simulink model "LoFT_Example3"  (R2024b)
settings: Solver=ode4  StartTime=0.0  StopTime=300  FixedStep=simu.dt  RelTol=1e-3
undefined symbols (not defined in the file): body, circtime, Communication, D1, Delta, irkb, line, LoFT, p0, Pn, s, simu, trip_time, Turbwind, waves, wind
libraries: simulink x350, spsThreePhaseVIMeasurementLib x41, spsThreePhasePISectionLineLib x34, spsThreePhaseParallelRLCLoadLib x21, spsThreePhaseTransformerTwoWindingsLib x14, spsLoadFlowBusLib x10, spsThreePhaseDynamicLoadLib x9, spsSynchronousMachinepuStandardLib x7, spsExcitationSystemLib x7, spsSteamTurbineandGovernorLib x7, spsGenericPowerSystemStabilizerLib x7, spsMultiBandPowerSystemStabilizerLib x7
(part 45 of 49)

== system LoFT_Example3/FOWT System/Subsystem7/FOWT9/Aerodynamics and Local Control Systems/Local Control Systems/Subsystem2 ==
  GenTorq : Inport
  BldPitch : Inport  Port=2
  Constant3 : Constant  Value=-Controller.torqueMax
  Gain 1 : Gain  Gain=Controller.SPS_kb/deg2rad(30)
  Gain 2 : Gain  Gain=Controller.omegaMax
  Gain 3 : Gain  Gain=-Controller.SPS_kt/Controller.torqueMax
  Sum5 : Sum  Inputs=|+-
  Sum6 : Sum  Inputs=|+-
  Delta_omega_g : Outport
  wires:
  Sum6/1 -> Gain 2/1
  Gain 1/1 -> Sum6/1
  Constant3/1 -> Sum5/2
  Gain 3/1 -> Sum6/2
  Sum5/1 -> Gain 3/1
  Gain 2/1 -> Delta_omega_g/1
  BldPitch/1 -> Gain 1/1
  GenTorq/1 -> Sum5/1

== system LoFT_Example3/FOWT System/Subsystem7/FOWT9/Aerodynamics and Local Control Systems/Local Control Systems/wind speed estimator ==
  In1 : Inport
  Discrete Filter : DiscreteFilter  Numerator=Controller.F.Wind.b  Denominator=Controller.F.Wind.a  InitialStates=2000
  Out1 : Outport
  wires:
  Discrete Filter/1 -> Out1/1
  In1/1 -> Discrete Filter/1

== system LoFT_Example3/Onshore grid/Onshore Grid/Subsystem/SG1/Regulators1/Turbine  & Excitation Regulators Mac2 ==
  Pref : Inport
  Vref : Inport  Port=2
  Vd : Inport  Port=3
  Vq : Inport  Port=4
  w : Inport  Port=5
  Pe : Inport  Port=6
  Add : Sum  Inputs=+-
  Excitation System : spsExcitationSystemLib/Excitation System  tr=20e-3  reg=[ 300, 0.001 ]  exc=[ 1, 0 ]  tgr=[ 0, 0 ]  damp=[ 0.001, 0.1 ]  sat=[ 0, 0 ]  lim=[ -11.5, 11.5, 0 ]  v0=[1 1.43]
  STG : spsSteamTurbineandGovernorLib/Steam Turbine and Governor  gentype=Tandem-compound (single mass)  reg1="[ 20  0.05    0 ]"  reg2="[ 0.001  0.15 ]"  reg3="[ -0.1  0.1  0  4.496 ]"  N=60*50  turb1="[ 0  10   3.3   0.5   ]"  turb2="[   0   0.36    0.36   0.28   ]"  HA="[ 0.046  1.430  1.465   0.192 ]"  KA="[ 90.44  53.88  64.59   62.94  ]"  DA="[ 0.0115  0.3575  0.3663   0.0137  ]"  ini1=1  ini2=[0.779316,-31.4247]
  Stabilisateur : Subsystem
  Terminator : Terminator
  Terminator1 : Terminator
  Terminator2 : Terminator
  wref : Constant
  wref1 : Constant
  Pm : Outport  VectorParamsAs1DForOutWhenUnconnected=off
  Vf : Outport  Port=2  VectorParamsAs1DForOutWhenUnconnected=off
  wires:
  Stabilisateur/1(Stab) -> Excitation System/4
  Add/1 -> STG/4, Stabilisateur/3(dw)
  wref1/1 -> Add/2
  Vd/1 -> Excitation System/2
  Vq/1 -> Excitation System/3
  w/1 -> STG/3, Add/1
  wref/1 -> STG/1
  Vref/1 -> Excitation System/1
  Pref/1 -> STG/2
  Pe/1 -> Stabilisateur/2(Pe)
  Excitation System/1 -> Vf/1
  STG/4 -> Stabilisateur/1(Pm), Pm/1
  STG/3 -> Terminator/1
  STG/2 -> Terminator1/1
  STG/1 -> Terminator2/1

== system LoFT_Example3/Onshore grid/Onshore Grid/Subsystem/SG2/Regulators2/Turbine  & Excitation Regulators Mac2 ==
  Pref : Inport
  Vref : Inport  Port=2
  Vd : Inport  Port=3
  Vq : Inport  Port=4
  w : Inport  Port=5
  Pe : Inport  Port=6
  Add : Sum  Inputs=+-
  Add1 : Sum
  Excitation System : spsExcitationSystemLib/Excitation System  tr=20e-3  reg=[ 300, 0.001 ]  exc=[ 1, 0 ]  tgr=[ 0, 0 ]  damp=[ 0.001, 0.1 ]  sat=[ 0, 0 ]  lim=[ -11.5, 11.5, 0 ]  v0=[1 1.43]
  STG : spsSteamTurbineandGovernorLib/Steam Turbine and Governor  gentype=Tandem-compound (single mass)  reg1="[ 20  0.05    0 ]"  reg2="[ 0.001  0.15 ]"  reg3="[ -0.1  0.1  0  4.496 ]"  N=60*50  turb1="[ 0  10   3.3   0.5   ]"  turb2="[   0   0.36    0.36   0.28   ]"  HA="[ 0.046  1.430  1.465   0.192 ]"  KA="[ 90.44  53.88  64.59   62.94  ]"  DA="[ 0.0115  0.3575  0.3663   0.0137  ]"  ini1=0.54  ini2=[0.779316,-31.4247]
  Stabilisateur : Subsystem
  Terminator : Terminator
  Terminator1 : Terminator
  Terminator2 : Terminator
  wref : Constant
  wref1 : Constant
  Pm : Outport  VectorParamsAs1DForOutWhenUnconnected=off
  Vf : Outport  Port=2  VectorParamsAs1DForOutWhenUnconnected=off
  wires:
  Stabilisateur/1(Stab) -> Excitation System/4
  Add/1 -> STG/4, Stabilisateur/3(dw)
  wref1/1 -> Add/2
  Vd/1 -> Excitation System/2
  Vq/1 -> Excitation System/3
  w/1 -> STG/3, Add/1
  wref/1 -> STG/1
  Vref/1 -> Excitation System/1
  Pref/1 -> STG/2
  Pe/1 -> Stabilisateur/2(Pe)
  Excitation System/1 -> Vf/1
  STG/4 -> Stabilisateur/1(Pm), Add1/2
  STG/3 -> Terminator/1
  STG/2 -> Terminator1/1
  STG/1 -> Terminator2/1
  Add1/1 -> Pm/1

== system LoFT_Example3/Onshore grid/Onshore Grid/Subsystem/SG4/Regulators4/Turbine  & Excitation Regulators Mac2 ==
  Pref : Inport
  Vref : Inport  Port=2
  Vd : Inport  Port=3
  Vq : Inport  Port=4
  w : Inport  Port=5
  Pe : Inport  Port=6
  Add : Sum  Inputs=+-
  Add1 : Sum
  Excitation System : spsExcitationSystemLib/Excitation System  tr=20e-3  reg=[ 300, 0.001 ]  exc=[ 1, 0 ]  tgr=[ 0, 0 ]  damp=[ 0.001, 0.1 ]  sat=[ 0, 0 ]  lim=[ -11.5, 11.5, 0 ]  v0=[1 1.43]
  STG : spsSteamTurbineandGovernorLib/Steam Turbine and Governor  gentype=Tandem-compound (single mass)  reg1="[ 20  0.05    0 ]"  reg2="[ 0.001  0.15 ]"  reg3="[ -0.1  0.1  0  4.496 ]"  N=60*50  turb1="[ 0  10   3.3   0.5   ]"  turb2="[   0   0.36    0.36   0.28   ]"  HA="[ 0.046  1.430  1.465   0.192 ]"  KA="[ 90.44  53.88  64.59   62.94  ]"  DA="[ 0.0115  0.3575  0.3663   0.0137  ]"  ini1=0.54  ini2=[0.779316,-31.4247]
  Stabilisateur : Subsystem
  Terminator : Terminator
  Terminator1 : Terminator
  Terminator2 : Terminator
  wref : Constant
  wref1 : Constant
  Pm : Outport  VectorParamsAs1DForOutWhenUnconnected=off
  Vf : Outport  Port=2  VectorParamsAs1DForOutWhenUnconnected=off
  wires:
  Stabilisateur/1(Stab) -> Excitation System/4
  Add/1 -> STG/4, Stabilisateur/3(dw)
  wref1/1 -> Add/2
  Vd/1 -> Excitation System/2
  Vq/1 -> Excitation System/3
  w/1 -> STG/3, Add/1
  wref/1 -> STG/1
  Vref/1 -> Excitation System/1
  Pref/1 -> STG/2
  Pe/1 -> Stabilisateur/2(Pe)
  Excitation System/1 -> Vf/1
  STG/4 -> Stabilisateur/1(Pm), Add1/2
  STG/3 -> Terminator/1
  STG/2 -> Terminator1/1
  STG/1 -> Terminator2/1
  Add1/1 -> Pm/1

== system LoFT_Example3/Onshore grid/Onshore Grid/Subsystem/SG5/Regulators5/Turbine  & Excitation Regulators Mac2 ==
  Pref : Inport
  Vref : Inport  Port=2
  Vd : Inport  Port=3
  Vq : Inport  Port=4
  w : Inport  Port=5
  Pe : Inport  Port=6
  Add : Sum  Inputs=+-
  Excitation System : spsExcitationSystemLib/Excitation System  tr=20e-3  reg=[ 300, 0.001 ]  exc=[ 1, 0 ]  tgr=[ 0, 0 ]  damp=[ 0.001, 0.1 ]  sat=[ 0, 0 ]  lim=[ -11.5, 11.5, 0 ]  v0=[1 1.43]
  STG : spsSteamTurbineandGovernorLib/Steam Turbine and Governor  gentype=Tandem-compound (single mass)  reg1="[ 20  0.05    0 ]"  reg2="[ 0.001  0.15 ]"  reg3="[ -0.1  0.1  0  4.496 ]"  N=60*50  turb1="[ 0  10   3.3   0.5   ]"  turb2="[   0   0.36    0.36   0.28   ]"  HA="[ 0.046  1.430  1.465   0.192 ]"  KA="[ 90.44  53.88  64.59   62.94  ]"  DA="[ 0.0115  0.3575  0.3663   0.0137  ]"  ini1=0.508  ini2=[0.779316,-31.4247]
  Stabilisateur : Subsystem
  Terminator : Terminator
  Terminator1 : Terminator
  Terminator2 : Terminator
  wref : Constant
  wref1 : Constant
  Pm : Outport  VectorParamsAs1DForOutWhenUnconnected=off
  Vf : Outport  Port=2  VectorParamsAs1DForOutWhenUnconnected=off
  wires:
  Stabilisateur/1(Stab) -> Excitation System/4
  Add/1 -> STG/4, Stabilisateur/3(dw)
  wref1/1 -> Add/2
  Vd/1 -> Excitation System/2
  Vq/1 -> Excitation System/3
  w/1 -> STG/3, Add/1
  wref/1 -> STG/1
  Vref/1 -> Excitation System/1
  Pref/1 -> STG/2
  Pe/1 -> Stabilisateur/2(Pe)
  Excitation System/1 -> Vf/1
  STG/4 -> Stabilisateur/1(Pm), Pm/1
  STG/3 -> Terminator/1
  STG/2 -> Terminator1/1
  STG/1 -> Terminator2/1

== system LoFT_Example3/Onshore grid/Onshore Grid/Subsystem/SG6/Regulators6/Turbine  & Excitation Regulators Mac2 ==
  Pref : Inport
  Vref : Inport  Port=2
  Vd : Inport  Port=3
  Vq : Inport  Port=4
  w : Inport  Port=5
  Pe : Inport  Port=6
  Add : Sum  Inputs=+-
  Add1 : Sum
  Excitation System : spsExcitationSystemLib/Excitation System  tr=20e-3  reg=[ 300, 0.001 ]  exc=[ 1, 0 ]  tgr=[ 0, 0 ]  damp=[ 0.001, 0.1 ]  sat=[ 0, 0 ]  lim=[ -11.5, 11.5, 0 ]  v0=[1 1.43]
  STG : spsSteamTurbineandGovernorLib/Steam Turbine and Governor  gentype=Tandem-compound (single mass)  reg1="[ 20  0.05    0 ]"  reg2="[ 0.001  0.15 ]"  reg3="[ -0.1  0.1  0  4.496 ]"  N=60*50  turb1="[ 0  10   3.3   0.5   ]"  turb2="[   0   0.36    0.36   0.28   ]"  HA="[ 0.046  1.430  1.465   0.192 ]"  KA="[ 90.44  53.88  64.59   62.94  ]"  DA="[ 0.0115  0.3575  0.3663   0.0137  ]"  ini1=0.54  ini2=[0.779316,-31.4247]
  Stabilisateur : Subsystem
  Subsystem : Subsystem
  Terminator : Terminator
  Terminator1 : Terminator
  Terminator2 : Terminator
  wref : Constant
  wref1 : Constant
  Pm : Outport  VectorParamsAs1DForOutWhenUnconnected=off
  Vf : Outport  Port=2  VectorParamsAs1DForOutWhenUnconnected=off
  wires:
  Stabilisateur/1(Stab) -> Excitation System/4
  Add/1 -> STG/4, Stabilisateur/3(dw)
  wref1/1 -> Add/2
  Vd/1 -> Excitation System/2
  Vq/1 -> Excitation System/3
  w/1 -> Subsystem/2(<Rotor speed  wm  (pu)>), STG/3, Add/1
  wref/1 -> Subsystem/1(In1), STG/1
  Vref/1 -> Excitation System/1
  Pref/1 -> STG/2
  Pe/1 -> Stabilisateur/2(Pe)
  Excitation System/1 -> Vf/1
  STG/4 -> Stabilisateur/1(Pm), Add1/2
  STG/3 -> Terminator/1
  STG/2 -> Terminator1/1
  STG/1 -> Terminator2/1
  Subsystem/1(Out1) -> Add1/1
  Add1/1 -> Pm/1

== system LoFT_Example3/Onshore grid/Onshore Grid/Subsystem/SG8/Regulators8/Turbine  & Excitation Regulators Mac2 ==
  Pref : Inport
  Vref : Inport  Port=2
  Vd : Inport  Port=3
  Vq : Inport  Port=4
  w : Inport  Port=5
  Pe : Inport  Port=6
  Add : Sum  Inputs=+-
  Add1 : Sum
  Excitation System : spsExcitationSystemLib/Excitation System  tr=20e-3  reg=[ 300, 0.001 ]  exc=[ 1, 0 ]  tgr=[ 0, 0 ]  damp=[ 0.001, 0.1 ]  sat=[ 0, 0 ]  lim=[ -11.5, 11.5, 0 ]  v0=[1 1.43]
  STG : spsSteamTurbineandGovernorLib/Steam Turbine and Governor  gentype=Tandem-compound (single mass)  reg1="[ 20  0.05    0 ]"  reg2="[ 0.001  0.15 ]"  reg3="[ -0.1  0.1  0  4.496 ]"  N=60*50  turb1="[ 0  10   3.3   0.5   ]"  turb2="[   0   0.36    0.36   0.28   ]"  HA="[ 0.046  1.430  1.465   0.192 ]"  KA="[ 90.44  53.88  64.59   62.94  ]"  DA="[ 0.0115  0.3575  0.3663   0.0137  ]"  ini1=0.54  ini2=[0.779316,-31.4247]
  Stabilisateur : Subsystem
  Subsystem : Subsystem
  Terminator : Terminator
  Terminator1 : Terminator
  Terminator2 : Terminator
  wref : Constant
  wref1 : Constant
  Pm : Outport  VectorParamsAs1DForOutWhenUnconnected=off
  Vf : Outport  Port=2  VectorParamsAs1DForOutWhenUnconnected=off
  wires:
  Stabilisateur/1(Stab) -> Excitation System/4
  Add/1 -> STG/4, Stabilisateur/3(dw)
  wref1/1 -> Add/2
  Vd/1 -> Excitation System/2
  Vq/1 -> Excitation System/3
  w/1 -> Subsystem/2(<Rotor speed  wm  (pu)>), STG/3, Add/1
  wref/1 -> Subsystem/1(In1), STG/1
  Vref/1 -> Excitation System/1
  Pref/1 -> STG/2
  Pe/1 -> Stabilisateur/2(Pe)
  Excitation System/1 -> Vf/1
  STG/4 -> Stabilisateur/1(Pm), Add1/2
  STG/3 -> Terminator/1
  STG/2 -> Terminator1/1
  STG/1 -> Terminator2/1
  Subsystem/1(Out1) -> Add1/1
  Add1/1 -> Pm/1

== system LoFT_Example3/Onshore grid/Onshore Grid/Subsystem/SG9/Regulators9/Turbine  & Excitation Regulators Mac2 ==
  Pref : Inport
  Vref : Inport  Port=2
  Vd : Inport  Port=3
  Vq : Inport  Port=4
  w : Inport  Port=5
  Pe : Inport  Port=6
  Add : Sum  Inputs=+-
  Excitation System : spsExcitationSystemLib/Excitation System  tr=20e-3  reg=[ 300, 0.001 ]  exc=[ 1, 0 ]  tgr=[ 0, 0 ]  damp=[ 0.001, 0.1 ]  sat=[ 0, 0 ]  lim=[ -11.5, 11.5, 0 ]  v0=[1 1.43]
  STG : spsSteamTurbineandGovernorLib/Steam Turbine and Governor  gentype=Tandem-compound (single mass)  reg1="[ 20  0.05    0 ]"  reg2="[ 0.001  0.15 ]"  reg3="[ -0.1  0.1  0  4.496 ]"  N=60*50  turb1="[ 0  10   3.3   0.5   ]"  turb2="[   0   0.36    0.36   0.28   ]"  HA="[ 0.046  1.430  1.465   0.192 ]"  KA="[ 90.44  53.88  64.59   62.94  ]"  DA="[ 0.0115  0.3575  0.3663   0.0137  ]"  ini1=0.83  ini2=[0.779316,-31.4247]
  Stabilisateur : Subsystem
  Terminator : Terminator
  Terminator1 : Terminator
  Terminator2 : Terminator
  wref : Constant
  wref1 : Constant
  Pm : Outport  VectorParamsAs1DForOutWhenUnconnected=off
  Vf : Outport  Port=2  VectorParamsAs1DForOutWhenUnconnected=off
  wires:
  Stabilisateur/1(Stab) -> Excitation System/4
  Add/1 -> STG/4, Stabilisateur/3(dw)
  wref1/1 -> Add/2
  Vd/1 -> Excitation System/2
  Vq/1 -> Excitation System/3
  w/1 -> STG/3, Add/1
  wref/1 -> STG/1
  Vref/1 -> Excitation System/1
  Pref/1 -> STG/2
  Pe/1 -> Stabilisateur/2(Pe)
  Excitation System/1 -> Vf/1
  STG/4 -> Stabilisateur/1(Pm), Pm/1
  STG/3 -> Terminator/1
  STG/2 -> Terminator1/1
  STG/1 -> Terminator2/1

== system LoFT_Example3/FOWT System/Subsystem1/FOWT1/Aerodynamics and Local Control Systems/Local Control Systems/Subsystem1/Gain Scheduling ==
  In1 : Inport
  In3 : Inport  Port=2
  In2 : Inport  Port=3
  1-D Lookup Table1 : Lookup_n-D  NumberOfTableDimensions=1  BreakpointsForDimension1=Controller.R.PC_GS_angles  Table=Controller.R.PC_GS_KI  InternalRulePriority=Speed  RndMeth=Simplest
  1-D Lookup Table2 : Lookup_n-D  NumberOfTableDimensions=1  BreakpointsForDimension1=Controller.R.PC_GS_angles  Table=Controller.R.PC_GS_KP  InternalRulePriority=Speed  RndMeth=Simplest
  Add : Sum
  Add1 : Sum
  Constant1 : Constant  Value=90*pi/180
  Delay : Delay  DelayLength=1  InitialCondition=0
  Gain : Gain  Gain=simu.dt
  Product : Product
  Product1 : Product
  Saturation Dynamic : simulink/Discontinuities/Saturation Dynamic  OutMin=[]  OutMax=[]  OutDataTypeStr=Inherit: Same as second input  OutDataType=fixdt(1, 16)  OutScaling=2^-10  DoSatur=off
  Saturation1 : Saturate  UpperLimit=Controller.R.PC_GS_KI(end)  LowerLimit=Controller.R.PC_GS_KI(1)
  Saturation3 : Saturate  UpperLimit=Controller.R.PC_GS_KP(end)  LowerLimit=Controller.R.PC_GS_KP(1)
  Out1 : Outport
  wires:
  Product/1 -> Add1/1
  Add1/1 -> Out1/1
  Delay/1 -> Add/2
  Saturation Dynamic/1 -> Delay/1, Add1/2
  Constant1/1 -> Saturation Dynamic/1
  In3/1 -> Saturation Dynamic/3
  Add/1 -> Saturation Dynamic/2
  Gain/1 -> Add/1
  Product1/1 -> Gain/1
  Saturation1/1 -> Product1/2
  Saturation3/1 -> Product/2
  In1/1 -> Product1/1, Product/1
  In2/1 -> 1-D Lookup Table2/1, 1-D Lookup Table1/1
  1-D Lookup Table2/1 -> Saturation3/1
  1-D Lookup Table1/1 -> Saturation1/1

== system LoFT_Example3/FOWT System/Subsystem1/FOWT10/Aerodynamics and Local Control Systems/Local Control Systems/Subsystem1/Gain Scheduling ==
  In1 : Inport
  In3 : Inport  Port=2
  In2 : Inport  Port=3
  1-D Lookup Table1 : Lookup_n-D  NumberOfTableDimensions=1  BreakpointsForDimension1=Controller.R.PC_GS_angles  Table=Controller.R.PC_GS_KI  InternalRulePriority=Speed  RndMeth=Simplest
  1-D Lookup Table2 : Lookup_n-D  NumberOfTableDimensions=1  BreakpointsForDimension1=Controller.R.PC_GS_angles  Table=Controller.R.PC_GS_KP  InternalRulePriority=Speed  RndMeth=Simplest
  Add : Sum
  Add1 : Sum
  Constant1 : Constant  Value=90*pi/180
  Delay : Delay  DelayLength=1  InitialCondition=0
  Gain : Gain  Gain=simu.dt
  Product : Product
  Product1 : Product
  Saturation Dynamic : simulink/Discontinuities/Saturation Dynamic  OutMin=[]  OutMax=[]  OutDataTypeStr=Inherit: Same as second input  OutDataType=fixdt(1, 16)  OutScaling=2^-10  DoSatur=off
  Saturation1 : Saturate  UpperLimit=Controller.R.PC_GS_KI(end)  LowerLimit=Controller.R.PC_GS_KI(1)
  Saturation3 : Saturate  UpperLimit=Controller.R.PC_GS_KP(end)  LowerLimit=Controller.R.PC_GS_KP(1)
  Out1 : Outport
  wires:
  1-D Lookup Table1/1 -> Saturation1/1
  1-D Lookup Table2/1 -> Saturation3/1
  In2/1 -> 1-D Lookup Table1/1, 1-D Lookup Table2/1
  In1/1 -> Product/1, Product1/1
  Saturation3/1 -> Product/2
  Saturation1/1 -> Product1/2
  Product1/1 -> Gain/1
  Gain/1 -> Add/1
  Add/1 -> Saturation Dynamic/2
  In3/1 -> Saturation Dynamic/3
  Constant1/1 -> Saturation Dynamic/1
  Saturation Dynamic/1 -> Add1/2, Delay/1
  Delay/1 -> Add/2
  Add1/1 -> Out1/1
  Product/1 -> Add1/1

== system LoFT_Example3/FOWT System/Subsystem1/FOWT2/Aerodynamics and Local Control Systems/Local Control Systems/Subsystem1/Gain Scheduling ==
  In1 : Inport
  In3 : Inport  Port=2
  In2 : Inport  Port=3
  1-D Lookup Table1 : Lookup_n-D  NumberOfTableDimensions=1  BreakpointsForDimension1=Controller.R.PC_GS_angles  Table=Controller.R.PC_GS_KI  InternalRulePriority=Speed  RndMeth=Simplest
  1-D Lookup Table2 : Lookup_n-D  NumberOfTableDimensions=1  BreakpointsForDimension1=Controller.R.PC_GS_angles  Table=Controller.R.PC_GS_KP  InternalRulePriority=Speed  RndMeth=Simplest
  Add : Sum
  Add1 : Sum
  Constant1 : Constant  Value=90*pi/180
  Delay : Delay  DelayLength=1  InitialCondition=0
  Gain : Gain  Gain=simu.dt
  Product : Product
  Product1 : Product
  Saturation Dynamic : simulink/Discontinuities/Saturation Dynamic  OutMin=[]  OutMax=[]  OutDataTypeStr=Inherit: Same as second input  OutDataType=fixdt(1, 16)  OutScaling=2^-10  DoSatur=off
  Saturation1 : Saturate  UpperLimit=Controller.R.PC_GS_KI(end)  LowerLimit=Controller.R.PC_GS_KI(1)
  Saturation3 : Saturate  UpperLimit=Controller.R.PC_GS_KP(end)  LowerLimit=Controller.R.PC_GS_KP(1)
  Out1 : Outport
  wires:
  1-D Lookup Table1/1 -> Saturation1/1
  1-D Lookup Table2/1 -> Saturation3/1
  In2/1 -> 1-D Lookup Table1/1, 1-D Lookup Table2/1
  In1/1 -> Product/1, Product1/1
  Saturation3/1 -> Product/2
  Saturation1/1 -> Product1/2
  Product1/1 -> Gain/1
  Gain/1 -> Add/1
  Add/1 -> Saturation Dynamic/2
  In3/1 -> Saturation Dynamic/3
  Constant1/1 -> Saturation Dynamic/1
  Saturation Dynamic/1 -> Add1/2, Delay/1
  Delay/1 -> Add/2
  Add1/1 -> Out1/1
  Product/1 -> Add1/1

== system LoFT_Example3/FOWT System/Subsystem1/FOWT3/Aerodynamics and Local Control Systems/Local Control Systems/Subsystem1/Gain Scheduling ==
  In1 : Inport
  In3 : Inport  Port=2
  In2 : Inport  Port=3
  1-D Lookup Table1 : Lookup_n-D  NumberOfTableDimensions=1  BreakpointsForDimension1=Controller.R.PC_GS_angles  Table=Controller.R.PC_GS_KI  InternalRulePriority=Speed  RndMeth=Simplest
  1-D Lookup Table2 : Lookup_n-D  NumberOfTableDimensions=1  BreakpointsForDimension1=Controller.R.PC_GS_angles  Table=Controller.R.PC_GS_KP  InternalRulePriority=Speed  RndMeth=Simplest
  Add : Sum
  Add1 : Sum
  Constant1 : Constant  Value=90*pi/180
  Delay : Delay  DelayLength=1  InitialCondition=0
  Gain : Gain  Gain=simu.dt
  Product : Product
  Product1 : Product
  Saturation Dynamic : simulink/Discontinuities/Saturation Dynamic  OutMin=[]  OutMax=[]  OutDataTypeStr=Inherit: Same as second input  OutDataType=fixdt(1, 16)  OutScaling=2^-10  DoSatur=off
  Saturation1 : Saturate  UpperLimit=Controller.R.PC_GS_KI(end)  LowerLimit=Controller.R.PC_GS_KI(1)
  Saturation3 : Saturate  UpperLimit=Controller.R.PC_GS_KP(end)  LowerLimit=Controller.R.PC_GS_KP(1)
  Out1 : Outport
  wires:
  Product/1 -> Add1/1
  Add1/1 -> Out1/1
  Delay/1 -> Add/2
  Saturation Dynamic/1 -> Delay/1, Add1/2
  Constant1/1 -> Saturation Dynamic/1
  In3/1 -> Saturation Dynamic/3
  Add/1 -> Saturation Dynamic/2
  Gain/1 -> Add/1
  Product1/1 -> Gain/1
  Saturation1/1 -> Product1/2
  Saturation3/1 -> Product/2
  In1/1 -> Product1/1, Product/1
  In2/1 -> 1-D Lookup Table2/1, 1-D Lookup Table1/1
  1-D Lookup Table2/1 -> Saturation3/1
  1-D Lookup Table1/1 -> Saturation1/1

== system LoFT_Example3/FOWT System/Subsystem1/FOWT4/Aerodynamics and Local Control Systems/Local Control Systems/Subsystem1/Gain Scheduling ==
  In1 : Inport
  In3 : Inport  Port=2
  In2 : Inport  Port=3
  1-D Lookup Table1 : Lookup_n-D  NumberOfTableDimensions=1  BreakpointsForDimension1=Controller.R.PC_GS_angles  Table=Controller.R.PC_GS_KI  InternalRulePriority=Speed  RndMeth=Simplest
  1-D Lookup Table2 : Lookup_n-D  NumberOfTableDimensions=1  BreakpointsForDimension1=Controller.R.PC_GS_angles  Table=Controller.R.PC_GS_KP  InternalRulePriority=Speed  RndMeth=Simplest
  Add : Sum
  Add1 : Sum
  Constant1 : Constant  Value=90*pi/180
  Delay : Delay  DelayLength=1  InitialCondition=0
  Gain : Gain  Gain=simu.dt
  Product : Product
  Product1 : Product
  Saturation Dynamic : simulink/Discontinuities/Saturation Dynamic  OutMin=[]  OutMax=[]  OutDataTypeStr=Inherit: Same as second input  OutDataType=fixdt(1, 16)  OutScaling=2^-10  DoSatur=off
  Saturation1 : Saturate  UpperLimit=Controller.R.PC_GS_KI(end)  LowerLimit=Controller.R.PC_GS_KI(1)
  Saturation3 : Saturate  UpperLimit=Controller.R.PC_GS_KP(end)  LowerLimit=Controller.R.PC_GS_KP(1)
  Out1 : Outport
  wires:
  1-D Lookup Table1/1 -> Saturation1/1
  1-D Lookup Table2/1 -> Saturation3/1
  In2/1 -> 1-D Lookup Table1/1, 1-D Lookup Table2/1
  In1/1 -> Product/1, Product1/1
  Saturation3/1 -> Product/2
  Saturation1/1 -> Product1/2
  Product1/1 -> Gain/1
  Gain/1 -> Add/1
  Add/1 -> Saturation Dynamic/2
  In3/1 -> Saturation Dynamic/3
  Constant1/1 -> Saturation Dynamic/1
  Saturation Dynamic/1 -> Add1/2, Delay/1
  Delay/1 -> Add/2
  Add1/1 -> Out1/1
  Product/1 -> Add1/1

== system LoFT_Example3/FOWT System/Subsystem1/FOWT5/Aerodynamics and Local Control Systems/Local Control Systems/Subsystem1/Gain Scheduling ==
  In1 : Inport
  In3 : Inport  Port=2
  In2 : Inport  Port=3
  1-D Lookup Table1 : Lookup_n-D  NumberOfTableDimensions=1  BreakpointsForDimension1=Controller.R.PC_GS_angles  Table=Controller.R.PC_GS_KI  InternalRulePriority=Speed  RndMeth=Simplest
  1-D Lookup Table2 : Lookup_n-D  NumberOfTableDimensions=1  BreakpointsForDimension1=Controller.R.PC_GS_angles  Table=Controller.R.PC_GS_KP  InternalRulePriority=Speed  RndMeth=Simplest
  Add : Sum
  Add1 : Sum
  Constant1 : Constant  Value=90*pi/180
  Delay : Delay  DelayLength=1  InitialCondition=0
  Gain : Gain  Gain=simu.dt
  Product : Product
  Product1 : Product
  Saturation Dynamic : simulink/Discontinuities/Saturation Dynamic  OutMin=[]  OutMax=[]  OutDataTypeStr=Inherit: Same as second input  OutDataType=fixdt(1, 16)  OutScaling=2^-10  DoSatur=off
  Saturation1 : Saturate  UpperLimit=Controller.R.PC_GS_KI(end)  LowerLimit=Controller.R.PC_GS_KI(1)
  Saturation3 : Saturate  UpperLimit=Controller.R.PC_GS_KP(end)  LowerLimit=Controller.R.PC_GS_KP(1)
  Out1 : Outport
  wires:
  Product/1 -> Add1/1
  Add1/1 -> Out1/1
  Delay/1 -> Add/2
  Saturation Dynamic/1 -> Delay/1, Add1/2
  Constant1/1 -> Saturation Dynamic/1
  In3/1 -> Saturation Dynamic/3
  Add/1 -> Saturation Dynamic/2
  Gain/1 -> Add/1
  Product1/1 -> Gain/1
  Saturation1/1 -> Product1/2
  Saturation3/1 -> Product/2
  In1/1 -> Product1/1, Product/1
  In2/1 -> 1-D Lookup Table2/1, 1-D Lookup Table1/1
  1-D Lookup Table2/1 -> Saturation3/1
  1-D Lookup Table1/1 -> Saturation1/1

== system LoFT_Example3/FOWT System/Subsystem1/FOWT6/Aerodynamics and Local Control Systems/Local Control Systems/Subsystem1/Gain Scheduling ==
  In1 : Inport
  In3 : Inport  Port=2
  In2 : Inport  Port=3
  1-D Lookup Table1 : Lookup_n-D  NumberOfTableDimensions=1  BreakpointsForDimension1=Controller.R.PC_GS_angles  Table=Controller.R.PC_GS_KI  InternalRulePriority=Speed  RndMeth=Simplest
  1-D Lookup Table2 : Lookup_n-D  NumberOfTableDimensions=1  BreakpointsForDimension1=Controller.R.PC_GS_angles  Table=Controller.R.PC_GS_KP  InternalRulePriority=Speed  RndMeth=Simplest
  Add : Sum
  Add1 : Sum
  Constant1 : Constant  Value=90*pi/180
  Delay : Delay  DelayLength=1  InitialCondition=0
  Gain : Gain  Gain=simu.dt
  Product : Product
  Product1 : Product
  Saturation Dynamic : simulink/Discontinuities/Saturation Dynamic  OutMin=[]  OutMax=[]  OutDataTypeStr=Inherit: Same as second input  OutDataType=fixdt(1, 16)  OutScaling=2^-10  DoSatur=off
  Saturation1 : Saturate  UpperLimit=Controller.R.PC_GS_KI(end)  LowerLimit=Controller.R.PC_GS_KI(1)
  Saturation3 : Saturate  UpperLimit=Controller.R.PC_GS_KP(end)  LowerLimit=Controller.R.PC_GS_KP(1)
  Out1 : Outport
  wires:
  1-D Lookup Table1/1 -> Saturation1/1
  1-D Lookup Table2/1 -> Saturation3/1
  In2/1 -> 1-D Lookup Table1/1, 1-D Lookup Table2/1
  In1/1 -> Product/1, Product1/1
  Saturation3/1 -> Product/2
  Saturation1/1 -> Product1/2
  Product1/1 -> Gain/1
  Gain/1 -> Add/1
  Add/1 -> Saturation Dynamic/2
  In3/1 -> Saturation Dynamic/3
  Constant1/1 -> Saturation Dynamic/1
  Saturation Dynamic/1 -> Add1/2, Delay/1
  Delay/1 -> Add/2
  Add1/1 -> Out1/1
  Product/1 -> Add1/1

== system LoFT_Example3/FOWT System/Subsystem1/FOWT7/Aerodynamics and Local Control Systems/Local Control Systems/Subsystem1/Gain Scheduling ==
  In1 : Inport
  In3 : Inport  Port=2
  In2 : Inport  Port=3
  1-D Lookup Table1 : Lookup_n-D  NumberOfTableDimensions=1  BreakpointsForDimension1=Controller.R.PC_GS_angles  Table=Controller.R.PC_GS_KI  InternalRulePriority=Speed  RndMeth=Simplest
  1-D Lookup Table2 : Lookup_n-D  NumberOfTableDimensions=1  BreakpointsForDimension1=Controller.R.PC_GS_angles  Table=Controller.R.PC_GS_KP  InternalRulePriority=Speed  RndMeth=Simplest
  Add : Sum
  Add1 : Sum
  Constant1 : Constant  Value=90*pi/180
  Delay : Delay  DelayLength=1  InitialCondition=0
  Gain : Gain  Gain=simu.dt
  Product : Product
  Product1 : Product
  Saturation Dynamic : simulink/Discontinuities/Saturation Dynamic  OutMin=[]  OutMax=[]  OutDataTypeStr=Inherit: Same as second input  OutDataType=fixdt(1, 16)  OutScaling=2^-10  DoSatur=off
  Saturation1 : Saturate  UpperLimit=Controller.R.PC_GS_KI(end)  LowerLimit=Controller.R.PC_GS_KI(1)
  Saturation3 : Saturate  UpperLimit=Controller.R.PC_GS_KP(end)  LowerLimit=Controller.R.PC_GS_KP(1)
  Out1 : Outport
  wires:
  Product/1 -> Add1/1
  Add1/1 -> Out1/1
  Delay/1 -> Add/2
  Saturation Dynamic/1 -> Delay/1, Add1/2
  Constant1/1 -> Saturation Dynamic/1
  In3/1 -> Saturation Dynamic/3
  Add/1 -> Saturation Dynamic/2
  Gain/1 -> Add/1
  Product1/1 -> Gain/1
  Saturation1/1 -> Product1/2
  Saturation3/1 -> Product/2
  In1/1 -> Product1/1, Product/1
  In2/1 -> 1-D Lookup Table2/1, 1-D Lookup Table1/1
  1-D Lookup Table2/1 -> Saturation3/1
  1-D Lookup Table1/1 -> Saturation1/1

== system LoFT_Example3/FOWT System/Subsystem1/FOWT8/Aerodynamics and Local Control Systems/Local Control Systems/Subsystem1/Gain Scheduling ==
  In1 : Inport
  In3 : Inport  Port=2
  In2 : Inport  Port=3
  1-D Lookup Table1 : Lookup_n-D  NumberOfTableDimensions=1  BreakpointsForDimension1=Controller.R.PC_GS_angles  Table=Controller.R.PC_GS_KI  InternalRulePriority=Speed  RndMeth=Simplest
  1-D Lookup Table2 : Lookup_n-D  NumberOfTableDimensions=1  BreakpointsForDimension1=Controller.R.PC_GS_angles  Table=Controller.R.PC_GS_KP  InternalRulePriority=Speed  RndMeth=Simplest
  Add : Sum
  Add1 : Sum
  Constant1 : Constant  Value=90*pi/180
  Delay : Delay  DelayLength=1  InitialCondition=0
  Gain : Gain  Gain=simu.dt
  Product : Product
  Product1 : Product
  Saturation Dynamic : simulink/Discontinuities/Saturation Dynamic  OutMin=[]  OutMax=[]  OutDataTypeStr=Inherit: Same as second input  OutDataType=fixdt(1, 16)  OutScaling=2^-10  DoSatur=off
  Saturation1 : Saturate  UpperLimit=Controller.R.PC_GS_KI(end)  LowerLimit=Controller.R.PC_GS_KI(1)
  Saturation3 : Saturate  UpperLimit=Controller.R.PC_GS_KP(end)  LowerLimit=Controller.R.PC_GS_KP(1)
  Out1 : Outport
  wires:
  1-D Lookup Table1/1 -> Saturation1/1
  1-D Lookup Table2/1 -> Saturation3/1
  In2/1 -> 1-D Lookup Table1/1, 1-D Lookup Table2/1
  In1/1 -> Product/1, Product1/1
  Saturation3/1 -> Product/2
  Saturation1/1 -> Product1/2
  Product1/1 -> Gain/1
  Gain/1 -> Add/1
  Add/1 -> Saturation Dynamic/2
  In3/1 -> Saturation Dynamic/3
  Constant1/1 -> Saturation Dynamic/1
  Saturation Dynamic/1 -> Add1/2, Delay/1
  Delay/1 -> Add/2
  Add1/1 -> Out1/1
  Product/1 -> Add1/1

== system LoFT_Example3/FOWT System/Subsystem1/FOWT9/Aerodynamics and Local Control Systems/Local Control Systems/Subsystem1/Gain Scheduling ==
  In1 : Inport
  In3 : Inport  Port=2
  In2 : Inport  Port=3
  1-D Lookup Table1 : Lookup_n-D  NumberOfTableDimensions=1  BreakpointsForDimension1=Controller.R.PC_GS_angles  Table=Controller.R.PC_GS_KI  InternalRulePriority=Speed  RndMeth=Simplest
  1-D Lookup Table2 : Lookup_n-D  NumberOfTableDimensions=1  BreakpointsForDimension1=Controller.R.PC_GS_angles  Table=Controller.R.PC_GS_KP  InternalRulePriority=Speed  RndMeth=Simplest
  Add : Sum
  Add1 : Sum
  Constant1 : Constant  Value=90*pi/180
  Delay : Delay  DelayLength=1  InitialCondition=0
  Gain : Gain  Gain=simu.dt
  Product : Product
  Product1 : Product
  Saturation Dynamic : simulink/Discontinuities/Saturation Dynamic  OutMin=[]  OutMax=[]  OutDataTypeStr=Inherit: Same as second input  OutDataType=fixdt(1, 16)  OutScaling=2^-10  DoSatur=off
  Saturation1 : Saturate  UpperLimit=Controller.R.PC_GS_KI(end)  LowerLimit=Controller.R.PC_GS_KI(1)
  Saturation3 : Saturate  UpperLimit=Controller.R.PC_GS_KP(end)  LowerLimit=Controller.R.PC_GS_KP(1)
  Out1 : Outport
  wires:
  Product/1 -> Add1/1
  Add1/1 -> Out1/1
  Delay/1 -> Add/2
  Saturation Dynamic/1 -> Delay/1, Add1/2
  Constant1/1 -> Saturation Dynamic/1
  In3/1 -> Saturation Dynamic/3
  Add/1 -> Saturation Dynamic/2
  Gain/1 -> Add/1
  Product1/1 -> Gain/1
  Saturation1/1 -> Product1/2
  Saturation3/1 -> Product/2
  In1/1 -> Product1/1, Product/1
  In2/1 -> 1-D Lookup Table2/1, 1-D Lookup Table1/1
  1-D Lookup Table2/1 -> Saturation3/1
  1-D Lookup Table1/1 -> Saturation1/1

== system LoFT_Example3/FOWT System/Subsystem11/FOWT1/Aerodynamics and Local Control Systems/Local Control Systems/Subsystem1/Gain Scheduling ==
  In1 : Inport
  In3 : Inport  Port=2
  In2 : Inport  Port=3
  1-D Lookup Table1 : Lookup_n-D  NumberOfTableDimensions=1  BreakpointsForDimension1=Controller.R.PC_GS_angles  Table=Controller.R.PC_GS_KI  InternalRulePriority=Speed  RndMeth=Simplest
  1-D Lookup Table2 : Lookup_n-D  NumberOfTableDimensions=1  BreakpointsForDimension1=Controller.R.PC_GS_angles  Table=Controller.R.PC_GS_KP  InternalRulePriority=Speed  RndMeth=Simplest
  Add : Sum
  Add1 : Sum
  Constant1 : Constant  Value=90*pi/180
  Delay : Delay  DelayLength=1  InitialCondition=0
  Gain : Gain  Gain=simu.dt
  Product : Product
  Product1 : Product
  Saturation Dynamic : simulink/Discontinuities/Saturation Dynamic  OutMin=[]  OutMax=[]  OutDataTypeStr=Inherit: Same as second input  OutDataType=fixdt(1, 16)  OutScaling=2^-10  DoSatur=off
  Saturation1 : Saturate  UpperLimit=Controller.R.PC_GS_KI(end)  LowerLimit=Controller.R.PC_GS_KI(1)
  Saturation3 : Saturate  UpperLimit=Controller.R.PC_GS_KP(end)  LowerLimit=Controller.R.PC_GS_KP(1)
  Out1 : Outport
  wires:
  Product/1 -> Add1/1
  Add1/1 -> Out1/1
  Delay/1 -> Add/2
  Saturation Dynamic/1 -> Delay/1, Add1/2
  Constant1/1 -> Saturation Dynamic/1
  In3/1 -> Saturation Dynamic/3
  Add/1 -> Saturation Dynamic/2
  Gain/1 -> Add/1
  Product1/1 -> Gain/1
  Saturation1/1 -> Product1/2
  Saturation3/1 -> Product/2
  In1/1 -> Product1/1, Product/1
  In2/1 -> 1-D Lookup Table2/1, 1-D Lookup Table1/1
  1-D Lookup Table2/1 -> Saturation3/1
  1-D Lookup Table1/1 -> Saturation1/1

== system LoFT_Example3/FOWT System/Subsystem11/FOWT10/Aerodynamics and Local Control Systems/Local Control Systems/Subsystem1/Gain Scheduling ==
  In1 : Inport
  In3 : Inport  Port=2
  In2 : Inport  Port=3
  1-D Lookup Table1 : Lookup_n-D  NumberOfTableDimensions=1  BreakpointsForDimension1=Controller.R.PC_GS_angles  Table=Controller.R.PC_GS_KI  InternalRulePriority=Speed  RndMeth=Simplest
  1-D Lookup Table2 : Lookup_n-D  NumberOfTableDimensions=1  BreakpointsForDimension1=Controller.R.PC_GS_angles  Table=Controller.R.PC_GS_KP  InternalRulePriority=Speed  RndMeth=Simplest
  Add : Sum
  Add1 : Sum
  Constant1 : Constant  Value=90*pi/180
  Delay : Delay  DelayLength=1  InitialCondition=0
  Gain : Gain  Gain=simu.dt
  Product : Product
  Product1 : Product
  Saturation Dynamic : simulink/Discontinuities/Saturation Dynamic  OutMin=[]  OutMax=[]  OutDataTypeStr=Inherit: Same as second input  OutDataType=fixdt(1, 16)  OutScaling=2^-10  DoSatur=off
  Saturation1 : Saturate  UpperLimit=Controller.R.PC_GS_KI(end)  LowerLimit=Controller.R.PC_GS_KI(1)
  Saturation3 : Saturate  UpperLimit=Controller.R.PC_GS_KP(end)  LowerLimit=Controller.R.PC_GS_KP(1)
  Out1 : Outport
  wires:
  1-D Lookup Table1/1 -> Saturation1/1
  1-D Lookup Table2/1 -> Saturation3/1
  In2/1 -> 1-D Lookup Table1/1, 1-D Lookup Table2/1
  In1/1 -> Product/1, Product1/1
  Saturation3/1 -> Product/2
  Saturation1/1 -> Product1/2
  Product1/1 -> Gain/1
  Gain/1 -> Add/1
  Add/1 -> Saturation Dynamic/2
  In3/1 -> Saturation Dynamic/3
  Constant1/1 -> Saturation Dynamic/1
  Saturation Dynamic/1 -> Add1/2, Delay/1
  Delay/1 -> Add/2
  Add1/1 -> Out1/1
  Product/1 -> Add1/1

== system LoFT_Example3/FOWT System/Subsystem11/FOWT2/Aerodynamics and Local Control Systems/Local Control Systems/Subsystem1/Gain Scheduling ==
  In1 : Inport
  In3 : Inport  Port=2
  In2 : Inport  Port=3
  1-D Lookup Table1 : Lookup_n-D  NumberOfTableDimensions=1  BreakpointsForDimension1=Controller.R.PC_GS_angles  Table=Controller.R.PC_GS_KI  InternalRulePriority=Speed  RndMeth=Simplest
  1-D Lookup Table2 : Lookup_n-D  NumberOfTableDimensions=1  BreakpointsForDimension1=Controller.R.PC_GS_angles  Table=Controller.R.PC_GS_KP  InternalRulePriority=Speed  RndMeth=Simplest
  Add : Sum
  Add1 : Sum
  Constant1 : Constant  Value=90*pi/180
  Delay : Delay  DelayLength=1  InitialCondition=0
  Gain : Gain  Gain=simu.dt
  Product : Product
  Product1 : Product
  Saturation Dynamic : simulink/Discontinuities/Saturation Dynamic  OutMin=[]  OutMax=[]  OutDataTypeStr=Inherit: Same as second input  OutDataType=fixdt(1, 16)  OutScaling=2^-10  DoSatur=off
  Saturation1 : Saturate  UpperLimit=Controller.R.PC_GS_KI(end)  LowerLimit=Controller.R.PC_GS_KI(1)
  Saturation3 : Saturate  UpperLimit=Controller.R.PC_GS_KP(end)  LowerLimit=Controller.R.PC_GS_KP(1)
  Out1 : Outport
  wires:
  1-D Lookup Table1/1 -> Saturation1/1
  1-D Lookup Table2/1 -> Saturation3/1
  In2/1 -> 1-D Lookup Table1/1, 1-D Lookup Table2/1
  In1/1 -> Product/1, Product1/1
  Saturation3/1 -> Product/2
  Saturation1/1 -> Product1/2
  Product1/1 -> Gain/1
  Gain/1 -> Add/1
  Add/1 -> Saturation Dynamic/2
  In3/1 -> Saturation Dynamic/3
  Constant1/1 -> Saturation Dynamic/1
  Saturation Dynamic/1 -> Add1/2, Delay/1
  Delay/1 -> Add/2
  Add1/1 -> Out1/1
  Product/1 -> Add1/1

== system LoFT_Example3/FOWT System/Subsystem11/FOWT3/Aerodynamics and Local Control Systems/Local Control Systems/Subsystem1/Gain Scheduling ==
  In1 : Inport
  In3 : Inport  Port=2
  In2 : Inport  Port=3
  1-D Lookup Table1 : Lookup_n-D  NumberOfTableDimensions=1  BreakpointsForDimension1=Controller.R.PC_GS_angles  Table=Controller.R.PC_GS_KI  InternalRulePriority=Speed  RndMeth=Simplest
  1-D Lookup Table2 : Lookup_n-D  NumberOfTableDimensions=1  BreakpointsForDimension1=Controller.R.PC_GS_angles  Table=Controller.R.PC_GS_KP  InternalRulePriority=Speed  RndMeth=Simplest
  Add : Sum
  Add1 : Sum
  Constant1 : Constant  Value=90*pi/180
  Delay : Delay  DelayLength=1  InitialCondition=0
  Gain : Gain  Gain=simu.dt
  Product : Product
  Product1 : Product
  Saturation Dynamic : simulink/Discontinuities/Saturation Dynamic  OutMin=[]  OutMax=[]  OutDataTypeStr=Inherit: Same as second input  OutDataType=fixdt(1, 16)  OutScaling=2^-10  DoSatur=off
  Saturation1 : Saturate  UpperLimit=Controller.R.PC_GS_KI(end)  LowerLimit=Controller.R.PC_GS_KI(1)
  Saturation3 : Saturate  UpperLimit=Controller.R.PC_GS_KP(end)  LowerLimit=Controller.R.PC_GS_KP(1)
  Out1 : Outport
  wires:
  Product/1 -> Add1/1
  Add1/1 -> Out1/1
  Delay/1 -> Add/2
  Saturation Dynamic/1 -> Delay/1, Add1/2
  Constant1/1 -> Saturation Dynamic/1
  In3/1 -> Saturation Dynamic/3
  Add/1 -> Saturation Dynamic/2
  Gain/1 -> Add/1
  Product1/1 -> Gain/1
  Saturation1/1 -> Product1/2
  Saturation3/1 -> Product/2
  In1/1 -> Product1/1, Product/1
  In2/1 -> 1-D Lookup Table2/1, 1-D Lookup Table1/1
  1-D Lookup Table2/1 -> Saturation3/1
  1-D Lookup Table1/1 -> Saturation1/1

== system LoFT_Example3/FOWT System/Subsystem11/FOWT4/Aerodynamics and Local Control Systems/Local Control Systems/Subsystem1/Gain Scheduling ==
  In1 : Inport
  In3 : Inport  Port=2
  In2 : Inport  Port=3
  1-D Lookup Table1 : Lookup_n-D  NumberOfTableDimensions=1  BreakpointsForDimension1=Controller.R.PC_GS_angles  Table=Controller.R.PC_GS_KI  InternalRulePriority=Speed  RndMeth=Simplest
  1-D Lookup Table2 : Lookup_n-D  NumberOfTableDimensions=1  BreakpointsForDimension1=Controller.R.PC_GS_angles  Table=Controller.R.PC_GS_KP  InternalRulePriority=Speed  RndMeth=Simplest
  Add : Sum
  Add1 : Sum
  Constant1 : Constant  Value=90*pi/180
  Delay : Delay  DelayLength=1  InitialCondition=0
  Gain : Gain  Gain=simu.dt
  Product : Product
  Product1 : Product
  Saturation Dynamic : simulink/Discontinuities/Saturation Dynamic  OutMin=[]  OutMax=[]  OutDataTypeStr=Inherit: Same as second input  OutDataType=fixdt(1, 16)  OutScaling=2^-10  DoSatur=off
  Saturation1 : Saturate  UpperLimit=Controller.R.PC_GS_KI(end)  LowerLimit=Controller.R.PC_GS_KI(1)
  Saturation3 : Saturate  UpperLimit=Controller.R.PC_GS_KP(end)  LowerLimit=Controller.R.PC_GS_KP(1)
  Out1 : Outport
  wires:
  1-D Lookup Table1/1 -> Saturation1/1
  1-D Lookup Table2/1 -> Saturation3/1
  In2/1 -> 1-D Lookup Table1/1, 1-D Lookup Table2/1
  In1/1 -> Product/1, Product1/1
  Saturation3/1 -> Product/2
  Saturation1/1 -> Product1/2
  Product1/1 -> Gain/1
  Gain/1 -> Add/1
  Add/1 -> Saturation Dynamic/2
  In3/1 -> Saturation Dynamic/3
  Constant1/1 -> Saturation Dynamic/1
  Saturation Dynamic/1 -> Add1/2, Delay/1
  Delay/1 -> Add/2
  Add1/1 -> Out1/1
  Product/1 -> Add1/1

== system LoFT_Example3/FOWT System/Subsystem11/FOWT5/Aerodynamics and Local Control Systems/Local Control Systems/Subsystem1/Gain Scheduling ==
  In1 : Inport
  In3 : Inport  Port=2
  In2 : Inport  Port=3
  1-D Lookup Table1 : Lookup_n-D  NumberOfTableDimensions=1  BreakpointsForDimension1=Controller.R.PC_GS_angles  Table=Controller.R.PC_GS_KI  InternalRulePriority=Speed  RndMeth=Simplest
  1-D Lookup Table2 : Lookup_n-D  NumberOfTableDimensions=1  BreakpointsForDimension1=Controller.R.PC_GS_angles  Table=Controller.R.PC_GS_KP  InternalRulePriority=Speed  RndMeth=Simplest
  Add : Sum
  Add1 : Sum
  Constant1 : Constant  Value=90*pi/180
  Delay : Delay  DelayLength=1  InitialCondition=0
  Gain : Gain  Gain=simu.dt
  Product : Product
  Product1 : Product
  Saturation Dynamic : simulink/Discontinuities/Saturation Dynamic  OutMin=[]  OutMax=[]  OutDataTypeStr=Inherit: Same as second input  OutDataType=fixdt(1, 16)  OutScaling=2^-10  DoSatur=off
  Saturation1 : Saturate  UpperLimit=Controller.R.PC_GS_KI(end)  LowerLimit=Controller.R.PC_GS_KI(1)
  Saturation3 : Saturate  UpperLimit=Controller.R.PC_GS_KP(end)  LowerLimit=Controller.R.PC_GS_KP(1)
  Out1 : Outport
  wires:
  Product/1 -> Add1/1
  Add1/1 -> Out1/1
  Delay/1 -> Add/2
  Saturation Dynamic/1 -> Delay/1, Add1/2
  Constant1/1 -> Saturation Dynamic/1
  In3/1 -> Saturation Dynamic/3
  Add/1 -> Saturation Dynamic/2
  Gain/1 -> Add/1
  Product1/1 -> Gain/1
  Saturation1/1 -> Product1/2
  Saturation3/1 -> Product/2
  In1/1 -> Product1/1, Product/1
  In2/1 -> 1-D Lookup Table2/1, 1-D Lookup Table1/1
  1-D Lookup Table2/1 -> Saturation3/1
  1-D Lookup Table1/1 -> Saturation1/1

== system LoFT_Example3/FOWT System/Subsystem11/FOWT6/Aerodynamics and Local Control Systems/Local Control Systems/Subsystem1/Gain Scheduling ==
  In1 : Inport
  In3 : Inport  Port=2
  In2 : Inport  Port=3
  1-D Lookup Table1 : Lookup_n-D  NumberOfTableDimensions=1  BreakpointsForDimension1=Controller.R.PC_GS_angles  Table=Controller.R.PC_GS_KI  InternalRulePriority=Speed  RndMeth=Simplest
  1-D Lookup Table2 : Lookup_n-D  NumberOfTableDimensions=1  BreakpointsForDimension1=Controller.R.PC_GS_angles  Table=Controller.R.PC_GS_KP  InternalRulePriority=Speed  RndMeth=Simplest
  Add : Sum
  Add1 : Sum
  Constant1 : Constant  Value=90*pi/180
  Delay : Delay  DelayLength=1  InitialCondition=0
  Gain : Gain  Gain=simu.dt
  Product : Product
  Product1 : Product
  Saturation Dynamic : simulink/Discontinuities/Saturation Dynamic  OutMin=[]  OutMax=[]  OutDataTypeStr=Inherit: Same as second input  OutDataType=fixdt(1, 16)  OutScaling=2^-10  DoSatur=off
  Saturation1 : Saturate  UpperLimit=Controller.R.PC_GS_KI(end)  LowerLimit=Controller.R.PC_GS_KI(1)
  Saturation3 : Saturate  UpperLimit=Controller.R.PC_GS_KP(end)  LowerLimit=Controller.R.PC_GS_KP(1)
  Out1 : Outport
  wires:
  1-D Lookup Table1/1 -> Saturation1/1
  1-D Lookup Table2/1 -> Saturation3/1
  In2/1 -> 1-D Lookup Table1/1, 1-D Lookup Table2/1
  In1/1 -> Product/1, Product1/1
  Saturation3/1 -> Product/2
  Saturation1/1 -> Product1/2
  Product1/1 -> Gain/1
  Gain/1 -> Add/1
  Add/1 -> Saturation Dynamic/2
  In3/1 -> Saturation Dynamic/3
  Constant1/1 -> Saturation Dynamic/1
  Saturation Dynamic/1 -> Add1/2, Delay/1
  Delay/1 -> Add/2
  Add1/1 -> Out1/1
  Product/1 -> Add1/1

== system LoFT_Example3/FOWT System/Subsystem11/FOWT7/Aerodynamics and Local Control Systems/Local Control Systems/Subsystem1/Gain Scheduling ==
  In1 : Inport
  In3 : Inport  Port=2
  In2 : Inport  Port=3
  1-D Lookup Table1 : Lookup_n-D  NumberOfTableDimensions=1  BreakpointsForDimension1=Controller.R.PC_GS_angles  Table=Controller.R.PC_GS_KI  InternalRulePriority=Speed  RndMeth=Simplest
  1-D Lookup Table2 : Lookup_n-D  NumberOfTableDimensions=1  BreakpointsForDimension1=Controller.R.PC_GS_angles  Table=Controller.R.PC_GS_KP  InternalRulePriority=Speed  RndMeth=Simplest
  Add : Sum
  Add1 : Sum
  Constant1 : Constant  Value=90*pi/180
  Delay : Delay  DelayLength=1  InitialCondition=0
  Gain : Gain  Gain=simu.dt
  Product : Product
  Product1 : Product
  Saturation Dynamic : simulink/Discontinuities/Saturation Dynamic  OutMin=[]  OutMax=[]  OutDataTypeStr=Inherit: Same as second input  OutDataType=fixdt(1, 16)  OutScaling=2^-10  DoSatur=off
  Saturation1 : Saturate  UpperLimit=Controller.R.PC_GS_KI(end)  LowerLimit=Controller.R.PC_GS_KI(1)
  Saturation3 : Saturate  UpperLimit=Controller.R.PC_GS_KP(end)  LowerLimit=Controller.R.PC_GS_KP(1)
  Out1 : Outport
  wires:
  Product/1 -> Add1/1
  Add1/1 -> Out1/1
  Delay/1 -> Add/2
  Saturation Dynamic/1 -> Delay/1, Add1/2
  Constant1/1 -> Saturation Dynamic/1
  In3/1 -> Saturation Dynamic/3
  Add/1 -> Saturation Dynamic/2
  Gain/1 -> Add/1
  Product1/1 -> Gain/1
  Saturation1/1 -> Product1/2
  Saturation3/1 -> Product/2
  In1/1 -> Product1/1, Product/1
  In2/1 -> 1-D Lookup Table2/1, 1-D Lookup Table1/1
  1-D Lookup Table2/1 -> Saturation3/1
  1-D Lookup Table1/1 -> Saturation1/1

== system LoFT_Example3/FOWT System/Subsystem11/FOWT8/Aerodynamics and Local Control Systems/Local Control Systems/Subsystem1/Gain Scheduling ==
  In1 : Inport
  In3 : Inport  Port=2
  In2 : Inport  Port=3
  1-D Lookup Table1 : Lookup_n-D  NumberOfTableDimensions=1  BreakpointsForDimension1=Controller.R.PC_GS_angles  Table=Controller.R.PC_GS_KI  InternalRulePriority=Speed  RndMeth=Simplest
  1-D Lookup Table2 : Lookup_n-D  NumberOfTableDimensions=1  BreakpointsForDimension1=Controller.R.PC_GS_angles  Table=Controller.R.PC_GS_KP  InternalRulePriority=Speed  RndMeth=Simplest
  Add : Sum
  Add1 : Sum
  Constant1 : Constant  Value=90*pi/180
  Delay : Delay  DelayLength=1  InitialCondition=0
  Gain : Gain  Gain=simu.dt
  Product : Product
  Product1 : Product
  Saturation Dynamic : simulink/Discontinuities/Saturation Dynamic  OutMin=[]  OutMax=[]  OutDataTypeStr=Inherit: Same as second input  OutDataType=fixdt(1, 16)  OutScaling=2^-10  DoSatur=off
  Saturation1 : Saturate  UpperLimit=Controller.R.PC_GS_KI(end)  LowerLimit=Controller.R.PC_GS_KI(1)
  Saturation3 : Saturate  UpperLimit=Controller.R.PC_GS_KP(end)  LowerLimit=Controller.R.PC_GS_KP(1)
  Out1 : Outport
  wires:
  1-D Lookup Table1/1 -> Saturation1/1
  1-D Lookup Table2/1 -> Saturation3/1
  In2/1 -> 1-D Lookup Table1/1, 1-D Lookup Table2/1
  In1/1 -> Product/1, Product1/1
  Saturation3/1 -> Product/2
  Saturation1/1 -> Product1/2
  Product1/1 -> Gain/1
  Gain/1 -> Add/1
  Add/1 -> Saturation Dynamic/2
  In3/1 -> Saturation Dynamic/3
  Constant1/1 -> Saturation Dynamic/1
  Saturation Dynamic/1 -> Add1/2, Delay/1
  Delay/1 -> Add/2
  Add1/1 -> Out1/1
  Product/1 -> Add1/1

== system LoFT_Example3/FOWT System/Subsystem11/FOWT9/Aerodynamics and Local Control Systems/Local Control Systems/Subsystem1/Gain Scheduling ==
  In1 : Inport
  In3 : Inport  Port=2
  In2 : Inport  Port=3
  1-D Lookup Table1 : Lookup_n-D  NumberOfTableDimensions=1  BreakpointsForDimension1=Controller.R.PC_GS_angles  Table=Controller.R.PC_GS_KI  InternalRulePriority=Speed  RndMeth=Simplest
  1-D Lookup Table2 : Lookup_n-D  NumberOfTableDimensions=1  BreakpointsForDimension1=Controller.R.PC_GS_angles  Table=Controller.R.PC_GS_KP  InternalRulePriority=Speed  RndMeth=Simplest
  Add : Sum
  Add1 : Sum
  Constant1 : Constant  Value=90*pi/180
  Delay : Delay  DelayLength=1  InitialCondition=0
  Gain : Gain  Gain=simu.dt
  Product : Product
  Product1 : Product
  Saturation Dynamic : simulink/Discontinuities/Saturation Dynamic  OutMin=[]  OutMax=[]  OutDataTypeStr=Inherit: Same as second input  OutDataType=fixdt(1, 16)  OutScaling=2^-10  DoSatur=off
  Saturation1 : Saturate  UpperLimit=Controller.R.PC_GS_KI(end)  LowerLimit=Controller.R.PC_GS_KI(1)
  Saturation3 : Saturate  UpperLimit=Controller.R.PC_GS_KP(end)  LowerLimit=Controller.R.PC_GS_KP(1)
  Out1 : Outport
  wires:
  Product/1 -> Add1/1
  Add1/1 -> Out1/1
  Delay/1 -> Add/2
  Saturation Dynamic/1 -> Delay/1, Add1/2
  Constant1/1 -> Saturation Dynamic/1
  In3/1 -> Saturation Dynamic/3
  Add/1 -> Saturation Dynamic/2
  Gain/1 -> Add/1
  Product1/1 -> Gain/1
  Saturation1/1 -> Product1/2
  Saturation3/1 -> Product/2
  In1/1 -> Product1/1, Product/1
  In2/1 -> 1-D Lookup Table2/1, 1-D Lookup Table1/1
  1-D Lookup Table2/1 -> Saturation3/1
  1-D Lookup Table1/1 -> Saturation1/1

== system LoFT_Example3/FOWT System/Subsystem13/FOWT1/Aerodynamics and Local Control Systems/Local Control Systems/Subsystem1/Gain Scheduling ==
  In1 : Inport
  In3 : Inport  Port=2
  In2 : Inport  Port=3
  1-D Lookup Table1 : Lookup_n-D  NumberOfTableDimensions=1  BreakpointsForDimension1=Controller.R.PC_GS_angles  Table=Controller.R.PC_GS_KI  InternalRulePriority=Speed  RndMeth=Simplest
  1-D Lookup Table2 : Lookup_n-D  NumberOfTableDimensions=1  BreakpointsForDimension1=Controller.R.PC_GS_angles  Table=Controller.R.PC_GS_KP  InternalRulePriority=Speed  RndMeth=Simplest
  Add : Sum
  Add1 : Sum
  Constant1 : Constant  Value=90*pi/180
  Delay : Delay  DelayLength=1  InitialCondition=0
  Gain : Gain  Gain=simu.dt
  Product : Product
  Product1 : Product
  Saturation Dynamic : simulink/Discontinuities/Saturation Dynamic  OutMin=[]  OutMax=[]  OutDataTypeStr=Inherit: Same as second input  OutDataType=fixdt(1, 16)  OutScaling=2^-10  DoSatur=off
  Saturation1 : Saturate  UpperLimit=Controller.R.PC_GS_KI(end)  LowerLimit=Controller.R.PC_GS_KI(1)
  Saturation3 : Saturate  UpperLimit=Controller.R.PC_GS_KP(end)  LowerLimit=Controller.R.PC_GS_KP(1)
  Out1 : Outport
  wires:
  1-D Lookup Table1/1 -> Saturation1/1
  1-D Lookup Table2/1 -> Saturation3/1
  In2/1 -> 1-D Lookup Table1/1, 1-D Lookup Table2/1
  In1/1 -> Product/1, Product1/1
  Saturation3/1 -> Product/2
  Saturation1/1 -> Product1/2
  Product1/1 -> Gain/1
  Gain/1 -> Add/1
  Add/1 -> Saturation Dynamic/2
  In3/1 -> Saturation Dynamic/3
  Constant1/1 -> Saturation Dynamic/1
  Saturation Dynamic/1 -> Add1/2, Delay/1
  Delay/1 -> Add/2
  Add1/1 -> Out1/1
  Product/1 -> Add1/1

== system LoFT_Example3/FOWT System/Subsystem13/FOWT10/Aerodynamics and Local Control Systems/Local Control Systems/Subsystem1/Gain Scheduling ==
  In1 : Inport
  In3 : Inport  Port=2
  In2 : Inport  Port=3
  1-D Lookup Table1 : Lookup_n-D  NumberOfTableDimensions=1  BreakpointsForDimension1=Controller.R.PC_GS_angles  Table=Controller.R.PC_GS_KI  InternalRulePriority=Speed  RndMeth=Simplest
  1-D Lookup Table2 : Lookup_n-D  NumberOfTableDimensions=1  BreakpointsForDimension1=Controller.R.PC_GS_angles  Table=Controller.R.PC_GS_KP  InternalRulePriority=Speed  RndMeth=Simplest
  Add : Sum
  Add1 : Sum
  Constant1 : Constant  Value=90*pi/180
  Delay : Delay  DelayLength=1  InitialCondition=0
  Gain : Gain  Gain=simu.dt
  Product : Product
  Product1 : Product
  Saturation Dynamic : simulink/Discontinuities/Saturation Dynamic  OutMin=[]  OutMax=[]  OutDataTypeStr=Inherit: Same as second input  OutDataType=fixdt(1, 16)  OutScaling=2^-10  DoSatur=off
  Saturation1 : Saturate  UpperLimit=Controller.R.PC_GS_KI(end)  LowerLimit=Controller.R.PC_GS_KI(1)
  Saturation3 : Saturate  UpperLimit=Controller.R.PC_GS_KP(end)  LowerLimit=Controller.R.PC_GS_KP(1)
  Out1 : Outport
  wires:
  Product/1 -> Add1/1
  Add1/1 -> Out1/1
  Delay/1 -> Add/2
  Saturation Dynamic/1 -> Delay/1, Add1/2
  Constant1/1 -> Saturation Dynamic/1
  In3/1 -> Saturation Dynamic/3
  Add/1 -> Saturation Dynamic/2
  Gain/1 -> Add/1
  Product1/1 -> Gain/1
  Saturation1/1 -> Product1/2
  Saturation3/1 -> Product/2
  In1/1 -> Product1/1, Product/1
  In2/1 -> 1-D Lookup Table2/1, 1-D Lookup Table1/1
  1-D Lookup Table2/1 -> Saturation3/1
  1-D Lookup Table1/1 -> Saturation1/1
